simulink model "jellystone_v2"  (R2016b)
settings: Solver=FixedStepAuto  StartTime=0.0  StopTime=1000  FixedStep=.1  RelTol=1e-3
settings Model: Creator=thomaskennedy  LastModifiedBy=thomaskennedy

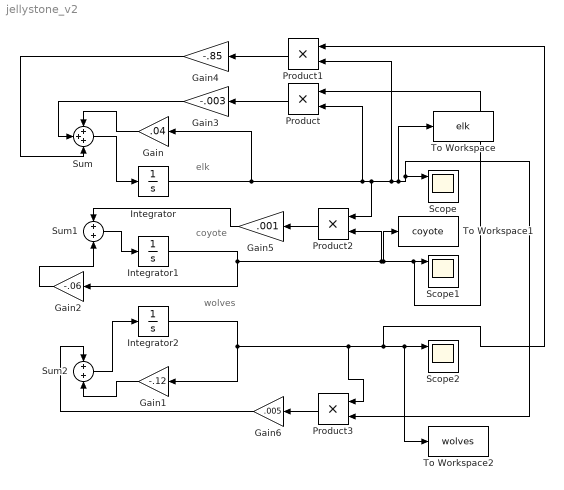
== system jellystone_v2 ==
  note: elk
  note: coyote
  note: wolves
  Gain : Gain  Gain=.04
  Gain1 : Gain  Gain=-.12
  Gain2 : Gain  Gain=-.06
  Gain3 : Gain  Gain=-.003
  Gain4 : Gain  Gain=-.85
  Gain5 : Gain  Gain=.001
  Gain6 : Gain  Gain=.005
  Integrator : Integrator  InitialCondition=31.217
  Integrator1 : Integrator  InitialCondition=2.017
  Integrator2 : Integrator  InitialCondition=[.001:.001:.03]
  Product{,1..3} (4 alike) : Product
  Scope : Scope  NumInputPorts=3
  Scope1 : Scope  NumInputPorts=3
  Scope2 : Scope  NumInputPorts=3
  Sum : Sum  Inputs=3
  Sum1 : Sum  Inputs=2
  Sum2 : Sum  Inputs=2
  To Workspace : ToWorkspace  VariableName=elk  SampleTime=-1
  To Workspace1 : ToWorkspace  VariableName=coyote  SampleTime=-1
  To Workspace2 : ToWorkspace  VariableName=wolves  SampleTime=-1
  wires:
  Integrator1/1 -> Gain2/1, Product2/2, Product/1, Scope1/1, To Workspace1/1
  Integrator2/1 -> Product3/1, Product1/1, To Workspace2/1, Scope2/1, Gain1/1
  Product/1 -> Gain3/1
  Gain/1 -> Sum/1
  Sum/1 -> Integrator/1
  Gain3/1 -> Sum/2
  Product1/1 -> Gain4/1
  Gain4/1 -> Sum/3
  Gain2/1 -> Sum1/2
  Sum1/1 -> Integrator1/1
  Product2/1 -> Gain5/1
  Gain5/1 -> Sum1/1
  Gain1/1 -> Sum2/2
  Sum2/1 -> Integrator2/1
  Integrator/1 -> Gain/1, Product/2, Product2/1, Product1/2, To Workspace/1, Product3/2, Scope/1
  Product3/1 -> Gain6/1
  Gain6/1 -> Sum2/1
